simulink model "New_Path_Following_with_Obstacle_Avoidance"  (R2021a)
settings: Solver=FixedStepAuto  StartTime=0.0  StopTime=inf  RelTol=1e-3
undefined symbols (not defined in the file): Angular, Linear, Sonar_Angels, waypoints
libraries: robotlib x5, robotalgslib x2
settings Model: Creator=tarun  LastModifiedBy=tarun
settings OptimizationCC: EnhancedBackFolding=on  PassReuseOutputArgsAs=Individual arguments  ZeroExternalMemoryAtStartup=off  ZeroInternalMemoryAtStartup=off  MaxStackSize=64  OptimizeBlockOrder=speed  DifferentSizesBufferReuse=on  OptimizationCustomize=off  EfficientTunableParamExpr=on
settings DebuggingCC: ParameterTunabilityLossMsg=error
settings HardwareCC: ProdBitPerPointer=32  ProdBitPerSizeT=32  ProdBitPerPtrDiffT=32  ProdLargestAtomicFloat=None  ProdIntDivRoundTo=Undefined  ProdEndianess=Unspecified  ProdWordSize=32  ProdHWDeviceType=Generic->Unspecified (assume 32-bit Generic)
settings SFSimCC: MATLABDynamicMemAlloc=off
settings RTWCC: SystemTargetFile=ert.tlc  HardwareBoard=Robot Operating System (ROS)  TLCOptions="-aInlineSetEventsForThisBaseRateFcn=TLC_FALSE -aSuppressMultiTaskScheduler=TLC_FALSE  -aRateBasedStepFcn=0"  TemplateMakefile=ert_default_tmf  Toolchain=Catkin  TargetLang=C++
settings CodeAppCC: ForceParamTrailComments=on  IgnoreCustomStorageClasses=off  OperatorAnnotations=on  SimulinkDataObjDesc=on  SFDataObjDesc=on  InsertBlockDesc=on
settings ERTTargetCC: SupportVariableSizeSignals=on

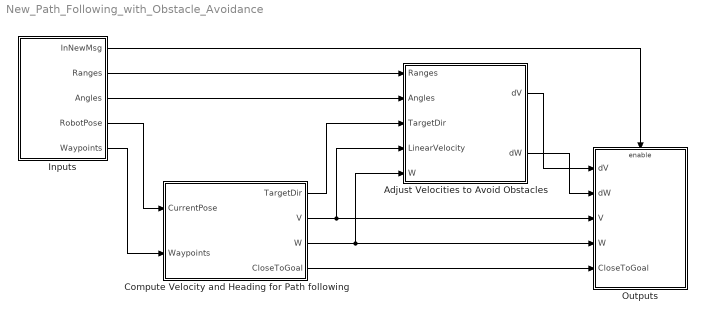
== system New_Path_Following_with_Obstacle_Avoidance ==
  Adjust Velocities to Avoid Obstacles : Subsystem
  Compute Velocity and Heading for Path following : Subsystem
  Inputs : Subsystem
  Outputs : Subsystem
  wires:
  Inputs/1(InNewMsg) -> Outputs/Enable
  Adjust Velocities to Avoid Obstacles/1(dV) -> Outputs/1(dV)
  Inputs/2(Ranges) -> Adjust Velocities to Avoid Obstacles/1(Ranges)
  Compute Velocity and Heading for Path following/1(TargetDir) -> Adjust Velocities to Avoid Obstacles/3(TargetDir)
  Compute Velocity and Heading for Path following/3(W) -> Adjust Velocities to Avoid Obstacles/5(W), Outputs/4(W)
  Compute Velocity and Heading for Path following/2(V) -> Adjust Velocities to Avoid Obstacles/4(LinearVelocity), Outputs/3(V)
  Inputs/5(Waypoints) -> Compute Velocity and Heading for Path following/2(Waypoints)
  Inputs/4(RobotPose) -> Compute Velocity and Heading for Path following/1(CurrentPose)
  Inputs/3(Angles) -> Adjust Velocities to Avoid Obstacles/2(Angles)
  Compute Velocity and Heading for Path following/4(CloseToGoal) -> Outputs/5(CloseToGoal)
  Adjust Velocities to Avoid Obstacles/2(dW) -> Outputs/2(dW)

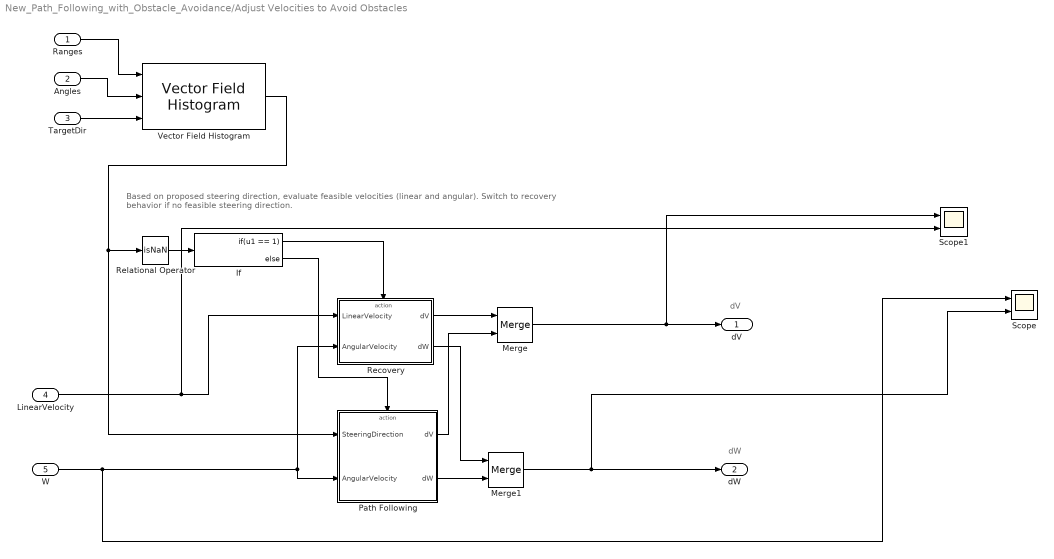
== system New_Path_Following_with_Obstacle_Avoidance/Adjust Velocities to Avoid Obstacles ==
  note: dV
  note: dW
  note: Based on proposed steering direction, evaluate feasible velocities (linear and angular).
      | 				Switch to recovery behavior if no feasible steering direction.
  Ranges : Inport
  Angles : Inport  Port=2
  TargetDir : Inport  Port=3
  LinearVelocity : Inport  Port=4
  W : Inport  Port=5
  If : If  IfExpression=u1 == 1
  Merge : Merge
  Merge1 : Merge
  Path Following : Subsystem  TreatAsAtomicUnit=on
  Recovery : Subsystem  TreatAsAtomicUnit=on
  Relational Operator : RelationalOperator  Operator=isNaN  OutDataTypeStr=boolean  RndMeth=Simplest
  Scope : Scope  NumInputPorts=2
  Scope1 : Scope  NumInputPorts=2
  Vector Field Histogram : robotalgslib/Vector Field Histogram  NumAngularSectors=84  DistanceLimits=[0.2,2]  HistogramThresholds=[1,2]  RobotRadius=0.475  SafetyDistance=0.2  MinTurningRadius=0.2  SimulateUsing=Code generation  TargetDirectionWeight=5  CurrentDirectionWeight=2  PreviousDirectionWeight=2
      settings: SourceProductBaseCode=NV,RO
  dV : Outport
  dW : Outport  Port=2
  wires:
  Angles/1 -> Vector Field Histogram/2
  TargetDir/1 -> Vector Field Histogram/3
  Ranges/1 -> Vector Field Histogram/1
  LinearVelocity/1 -> Scope1/2, Recovery/1(LinearVelocity)
  W/1 -> Scope/1, Path Following/2(AngularVelocity), Recovery/2(AngularVelocity)
  Path Following/1(dV) -> Merge/2
  Recovery/1(dV) -> Merge/1
  Merge/1 -> Scope1/1, dV/1
  Merge1/1 -> Scope/2, dW/1
  If/2 -> Path Following/Action
  Recovery/2(dW) -> Merge1/1
  Relational Operator/1 -> If/1
  If/1 -> Recovery/Action
  Vector Field Histogram/1 -> Path Following/1(SteeringDirection), Relational Operator/1
  Path Following/2(dW) -> Merge1/2

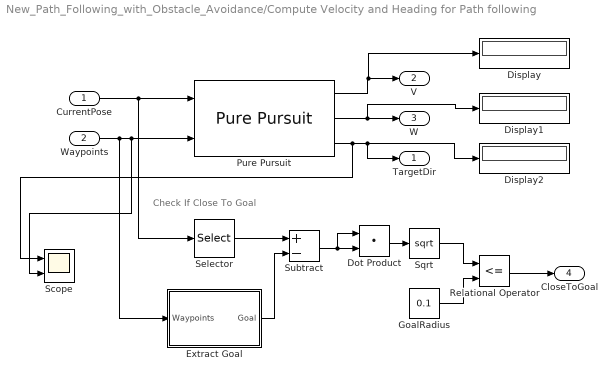
== system New_Path_Following_with_Obstacle_Avoidance/Compute Velocity and Heading for Path following ==
  note: Check If Close To Goal
  CurrentPose : Inport
  Waypoints : Inport  Port=2
  " Extract Goal" : MATLAB Function  TreatAsAtomicUnit=on
  Display : Display
  Display1 : Display
  Display2 : Display
  Dot Product : DotProduct  InputSameDT=on  OutDataTypeStr=Inherit: Inherit via internal rule
  GoalRadius : Constant  Value=0.1
  Pure Pursuit : robotalgslib/Pure Pursuit  DesiredLinearVelocity=0.3  MaxAngularVelocity=0.1  LookaheadDistance=0.45  TargetDirPort=on  SimulateUsing=Code generation
  Relational Operator : RelationalOperator  Operator=<=  OutDataTypeStr=boolean  RndMeth=Simplest
  Scope : Scope  NumInputPorts=2
  Selector : Selector  InputPortWidth=3  IndexOptions=Index vector (dialog)  Indices=[1 2]  OutputSizes=1
  Sqrt : Sqrt  SaturateOnIntegerOverflow=on
  Subtract : Sum  Inputs=+-
  TargetDir : Outport  VectorParamsAs1DForOutWhenUnconnected=off
  V : Outport  Port=2  VectorParamsAs1DForOutWhenUnconnected=off
  W : Outport  Port=3  VectorParamsAs1DForOutWhenUnconnected=off
  CloseToGoal : Outport  Port=4  VectorParamsAs1DForOutWhenUnconnected=off
  wires:
  Pure Pursuit/3 -> Scope/1, Display2/1, TargetDir/1
  Pure Pursuit/2 -> Display1/1, W/1
  Pure Pursuit/1 -> Display/1, V/1
  CurrentPose/1 -> Selector/1, Pure Pursuit/1
  Relational Operator/1 -> CloseToGoal/1
  GoalRadius/1 -> Relational Operator/2
  Selector/1 -> Subtract/1
  Dot Product/1 -> Sqrt/1
  Sqrt/1 -> Relational Operator/1
  Subtract/1 -> Dot Product/1, Dot Product/2
  " Extract Goal"/1(Goal) -> Subtract/2
  Waypoints/1 -> " Extract Goal"/1(Waypoints), Scope/2, Pure Pursuit/2

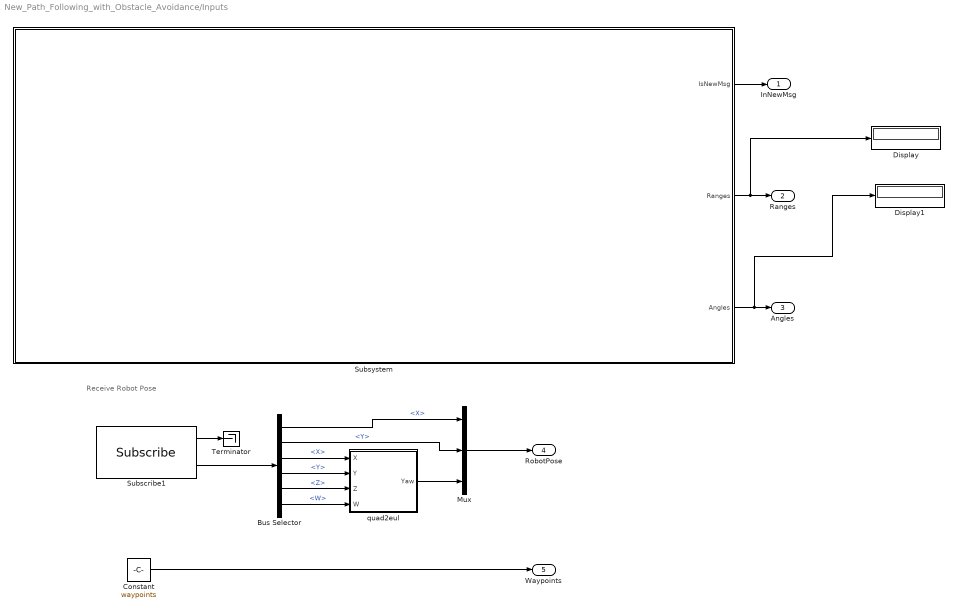
== system New_Path_Following_with_Obstacle_Avoidance/Inputs ==
  note: Receive Robot Pose
  Bus Selector : BusSelector  OutputSignals=Pose.Pose.Position.X,Pose.Pose.Position.Y,Pose.Pose.Orientation.X,Pose.Pose.Orientation.Y,Pose.Pose.Orientation.Z,Pose.Pose.Orientation.W
  Constant : Constant  Value=waypoints
  Display : Display
  Display1 : Display
  Mux : Mux  Inputs=3
  Subscribe1 : robotlib/Subscribe  topicSource=Specify your own  topic=/RosAria/pose  messageType=nav_msgs/Odometry  SampleTime=-1  legacyBusStruct=off  messageQueueLength=1
  Subsystem : Subsystem
  Terminator : Terminator
  quad2eul : MATLAB Function  TreatAsAtomicUnit=on
  InNewMsg : Outport
  Ranges : Outport  Port=2
  Angles : Outport  Port=3
  RobotPose : Outport  Port=4  VectorParamsAs1DForOutWhenUnconnected=off
  Waypoints : Outport  Port=5  VectorParamsAs1DForOutWhenUnconnected=off
  wires:
  quad2eul/1(Yaw) -> Mux/3
  Subscribe1/2 -> Bus Selector/1
  Bus Selector/3 -> quad2eul/1(X)  "<X>"
  Subscribe1/1 -> Terminator/1
  Bus Selector/2 -> Mux/2  "<Y>"
  Bus Selector/5 -> quad2eul/3(Z)  "<Z>"
  Bus Selector/4 -> quad2eul/2(Y)  "<Y>"
  Bus Selector/1 -> Mux/1  "<X>"
  Bus Selector/6 -> quad2eul/4(W)  "<W>"
  Mux/1 -> RobotPose/1
  Subsystem/3(Angles) -> Display1/1, Angles/1
  Subsystem/2(Ranges) -> Display/1, Ranges/1
  Subsystem/1(IsNewMsg) -> InNewMsg/1
  Constant/1 -> Waypoints/1

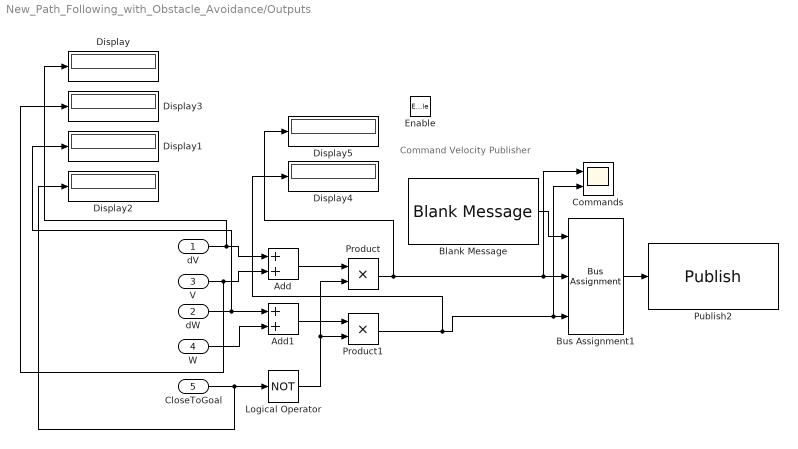
== system New_Path_Following_with_Obstacle_Avoidance/Outputs ==
  note: Command Velocity Publisher
  dV : Inport
  dW : Inport  Port=2
  V : Inport  Port=3
  W : Inport  Port=4
  CloseToGoal : Inport  Port=5
  Enable : EnablePort
  Add : Sum
  Add1 : Sum
  Blank Message : robotlib/Blank Message  messageClass=Message  entityType=geometry_msgs/Twist  messageType=geometry_msgs/Twist  SampleTime=inf  legacyBusStruct=off
  Bus Assignment1 : BusAssignment  DialogController=Simulink.DDGSource_BusAssignment  AssignedSignals=Linear.X,Angular.Z
  Commands : Scope  NumInputPorts=2
  Display{,1..5} (6 alike) : Display
  Logical Operator : Logic  Operator=NOT  AllPortsSameDT=off  OutDataTypeStr=boolean
  Product : Product
  Product1 : Product
  Publish2 : robotlib/Publish  topicSource=Select from ROS network  topic=/RosAria/cmd_vel  messageType=geometry_msgs/Twist  legacyBusStruct=off  messageQueueLength=105
  wires:
  V/1 -> Display3/1, Add/2
  W/1 -> Add1/2
  dV/1 -> Display/1, Add/1
  dW/1 -> Display1/1, Add1/1
  CloseToGoal/1 -> Display2/1, Logical Operator/1
  Add/1 -> Product/1
  Add1/1 -> Product1/1
  Product/1 -> Display5/1, Bus Assignment1/2, Commands/1
  Blank Message/1 -> Bus Assignment1/1
  Bus Assignment1/1 -> Publish2/1
  Logical Operator/1 -> Product1/2, Product/2
  Product1/1 -> Display4/1, Commands/2, Bus Assignment1/3

== system New_Path_Following_with_Obstacle_Avoidance/Adjust Velocities to Avoid Obstacles/Path Following ==
  SteeringDirection : Inport
  AngularVelocity : Inport  Port=2
  Action Port : ActionPort  ActionPortLabel=else
  Compute Angular Velocity : MATLAB Function  TreatAsAtomicUnit=on
  Constant : Constant  Value=0
  MaxAngularVelocity : Constant
  Subtract : Sum  Inputs=+-
  dV : Outport  VectorParamsAs1DForOutWhenUnconnected=off
  dW : Outport  Port=2  VectorParamsAs1DForOutWhenUnconnected=off
  wires:
  Constant/1 -> dV/1
  MaxAngularVelocity/1 -> Compute Angular Velocity/2(wMax)
  SteeringDirection/1 -> Compute Angular Velocity/1(steeringDir)
  Subtract/1 -> dW/1
  Compute Angular Velocity/1(w) -> Subtract/1
  AngularVelocity/1 -> Subtract/2

== system New_Path_Following_with_Obstacle_Avoidance/Adjust Velocities to Avoid Obstacles/Recovery ==
  LinearVelocity : Inport
  AngularVelocity : Inport  Port=2
  Action Port : ActionPort  ActionPortLabel=if(u1 == 1)
  Constant1 : Constant  Value=0.2
  Gain : Gain  Gain=-1
  Subtract : Sum  Inputs=+-
  dV : Outport  VectorParamsAs1DForOutWhenUnconnected=off
  dW : Outport  Port=2  VectorParamsAs1DForOutWhenUnconnected=off
  wires:
  LinearVelocity/1 -> Gain/1
  Gain/1 -> dV/1
  Constant1/1 -> Subtract/1
  AngularVelocity/1 -> Subtract/2
  Subtract/1 -> dW/1

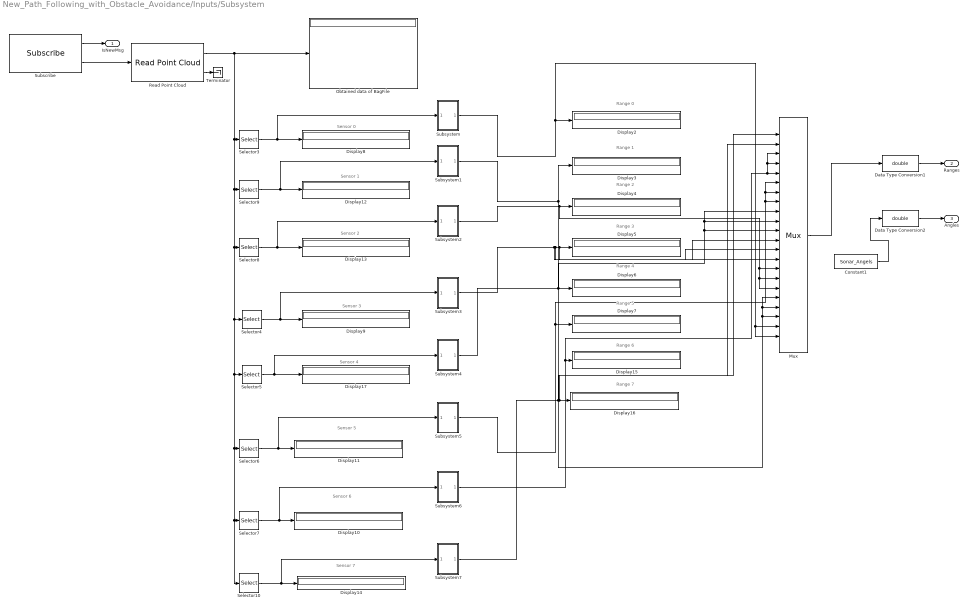
== system New_Path_Following_with_Obstacle_Avoidance/Inputs/Subsystem ==
  note: Range 7
  note: Range 4
  note: Sensor 2
  note: Range 2
  note: Sensor 3
  note: Sensor 1
  note: Range 3
  note: Sensor 6
  note: Range 5
  note: Range 0
  note: Sensor 0
  note: Sensor 4
  note: Sensor 5
  note: Range 1
  note: Range 6
  note: Sensor 7
  Constant1 : Constant  Value=Sonar_Angels
  Data Type Conversion1 : DataTypeConversion  OutDataTypeStr=double
  Data Type Conversion2 : DataTypeConversion  OutDataTypeStr=double
  Display{2..17} (16 alike) : Display
  Mux : Mux  Inputs=22
  Obtained data of BagFile : Display
  Read Point Cloud : robotlib/Read Point Cloud  MaximumPointCloudSize=[8, 1]  PreserveStructure=off  ShowRGBOutput=off  ShowIntensityOutput=off  ShowErrorCodeOutput=on  VariableSizeOutputs=off
      settings: SourceProductBaseCode=RR
  Selector10 : Selector  NumberOfDimensions=2  InputPortWidth=6  IndexOptions=Starting index (dialog),Starting index (dialog)  Indices=8,1  OutputSizes=1,3
  Selector3 : Selector  NumberOfDimensions=2  InputPortWidth=6  IndexOptions=Starting index (dialog),Starting index (dialog)  Indices=1,1  OutputSizes=1,3
  Selector4 : Selector  NumberOfDimensions=2  InputPortWidth=6  IndexOptions=Starting index (dialog),Starting index (dialog)  Indices=4,1  OutputSizes=1,3
  Selector5 : Selector  NumberOfDimensions=2  InputPortWidth=6  IndexOptions=Starting index (dialog),Starting index (dialog)  Indices=5,1  OutputSizes=1,3
  Selector6 : Selector  NumberOfDimensions=2  InputPortWidth=6  IndexOptions=Starting index (dialog),Starting index (dialog)  Indices=6,1  OutputSizes=1,3
  Selector7 : Selector  NumberOfDimensions=2  InputPortWidth=6  IndexOptions=Starting index (dialog),Starting index (dialog)  Indices=7,1  OutputSizes=1,3
  Selector8 : Selector  NumberOfDimensions=2  InputPortWidth=6  IndexOptions=Starting index (dialog),Starting index (dialog)  Indices=3,1  OutputSizes=1,3
  Selector9 : Selector  NumberOfDimensions=2  InputPortWidth=6  IndexOptions=Starting index (dialog),Starting index (dialog)  Indices=2,1  OutputSizes=1,3
  Subscribe : robotlib/Subscribe  topicSource=Select from ROS network  topic=/RosAria/sonar_pointcloud2  messageType=sensor_msgs/PointCloud2  SampleTime=0.05  legacyBusStruct=off  messageQueueLength=1
  Subsystem : Subsystem
  Subsystem1 : Subsystem
  Subsystem2 : Subsystem
  Subsystem3 : Subsystem
  Subsystem4 : Subsystem
  Subsystem5 : Subsystem
  Subsystem6 : Subsystem
  Subsystem7 : Subsystem
  Terminator : Terminator
  IsNewMsg : Outport
  Ranges : Outport  Port=2
  Angles : Outport  Port=3
  wires:
  Mux/1 -> Data Type Conversion1/1
  Constant1/1 -> Data Type Conversion2/1
  Selector4/1 -> Subsystem3/1(In1), Display9/1
  Subsystem7/1(Out1) -> Mux/2, Mux/1, Display16/1
  Selector8/1 -> Subsystem2/1(In1), Display13/1
  Subsystem5/1(Out1) -> Mux/6, Mux/7, Mux/8, Display7/1
  Selector9/1 -> Subsystem1/1(In1), Display12/1
  Subsystem2/1(Out1) -> Mux/17, Mux/16, Mux/15, Display4/1
  Selector3/1 -> Subsystem/1(In1), Display8/1
  Subsystem6/1(Out1) -> Mux/4, Mux/3, Mux/5, Display15/1
  Read Point Cloud/2 -> Terminator/1
  Subsystem4/1(Out1) -> Mux/9, Mux/10, Mux/11, Display6/1
  Selector6/1 -> Subsystem5/1(In1), Display11/1
  Subsystem1/1(Out1) -> Mux/20, Mux/19, Mux/18, Display3/1
  Subsystem/1(Out1) -> Mux/22, Mux/21, Display2/1
  Selector5/1 -> Subsystem4/1(In1), Display17/1
  Selector10/1 -> Subsystem7/1(In1), Display14/1
  Subsystem3/1(Out1) -> Mux/13, Mux/12, Mux/14, Display5/1
  Selector7/1 -> Subsystem6/1(In1), Display10/1
  Subscribe/2 -> Read Point Cloud/1
  Read Point Cloud/1 -> Obtained data of BagFile/1, Selector3/1, Selector9/1, Selector8/1, Selector4/1, Selector5/1, Selector6/1, Selector10/1, Selector7/1
  Subscribe/1 -> IsNewMsg/1
  Data Type Conversion1/1 -> Ranges/1
  Data Type Conversion2/1 -> Angles/1

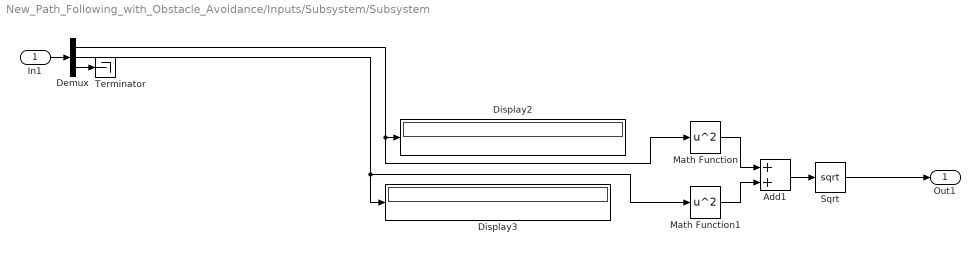
== system New_Path_Following_with_Obstacle_Avoidance/Inputs/Subsystem/Subsystem ==
  In1 : Inport
  Add1 : Sum
  Demux : Demux  Outputs=3
  Display2 : Display
  Display3 : Display
  Math Function : Math  Operator=square  SaturateOnIntegerOverflow=on
  Math Function1 : Math  Operator=square  SaturateOnIntegerOverflow=on
  Sqrt : Sqrt  SaturateOnIntegerOverflow=on
  Terminator : Terminator
  Out1 : Outport
  wires:
  Math Function1/1 -> Add1/2
  Demux/1 -> Math Function/1, Display2/1
  In1/1 -> Demux/1
  Math Function/1 -> Add1/1
  Demux/2 -> Display3/1, Math Function1/1
  Sqrt/1 -> Out1/1
  Add1/1 -> Sqrt/1
  Demux/3 -> Terminator/1

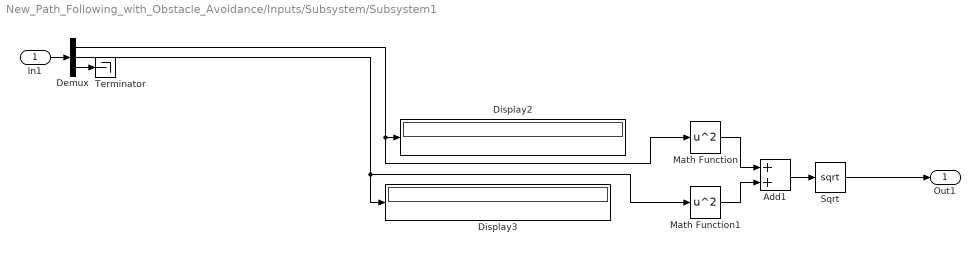
== system New_Path_Following_with_Obstacle_Avoidance/Inputs/Subsystem/Subsystem1 ==
  In1 : Inport
  Add1 : Sum
  Demux : Demux  Outputs=3
  Display2 : Display
  Display3 : Display
  Math Function : Math  Operator=square  SaturateOnIntegerOverflow=on
  Math Function1 : Math  Operator=square  SaturateOnIntegerOverflow=on
  Sqrt : Sqrt  SaturateOnIntegerOverflow=on
  Terminator : Terminator
  Out1 : Outport
  wires:
  Math Function1/1 -> Add1/2
  Demux/1 -> Math Function/1, Display2/1
  In1/1 -> Demux/1
  Math Function/1 -> Add1/1
  Demux/2 -> Display3/1, Math Function1/1
  Sqrt/1 -> Out1/1
  Add1/1 -> Sqrt/1
  Demux/3 -> Terminator/1

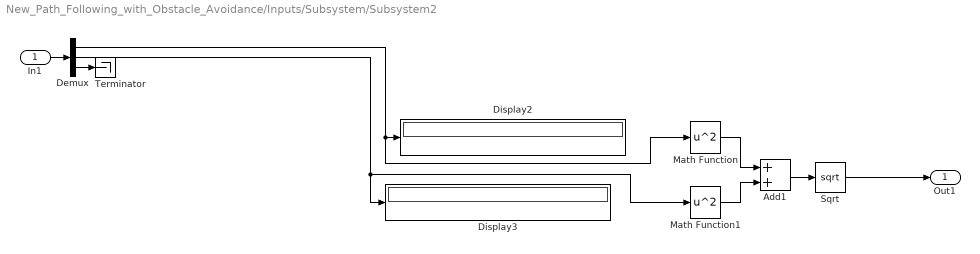
== system New_Path_Following_with_Obstacle_Avoidance/Inputs/Subsystem/Subsystem2 ==
  In1 : Inport
  Add1 : Sum
  Demux : Demux  Outputs=3
  Display2 : Display
  Display3 : Display
  Math Function : Math  Operator=square  SaturateOnIntegerOverflow=on
  Math Function1 : Math  Operator=square  SaturateOnIntegerOverflow=on
  Sqrt : Sqrt  SaturateOnIntegerOverflow=on
  Terminator : Terminator
  Out1 : Outport
  wires:
  Math Function1/1 -> Add1/2
  Demux/1 -> Math Function/1, Display2/1
  In1/1 -> Demux/1
  Math Function/1 -> Add1/1
  Demux/2 -> Display3/1, Math Function1/1
  Sqrt/1 -> Out1/1
  Add1/1 -> Sqrt/1
  Demux/3 -> Terminator/1

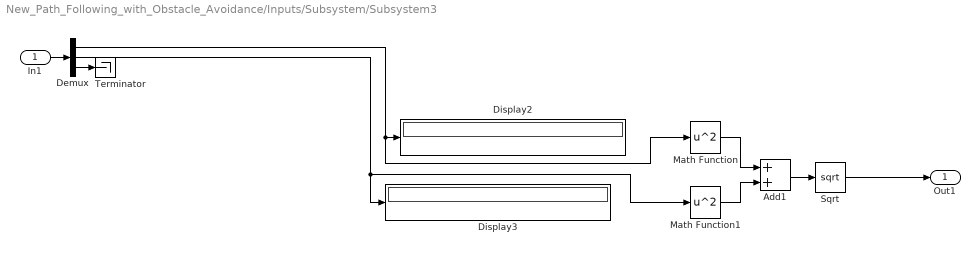
== system New_Path_Following_with_Obstacle_Avoidance/Inputs/Subsystem/Subsystem3 ==
  In1 : Inport
  Add1 : Sum
  Demux : Demux  Outputs=3
  Display2 : Display
  Display3 : Display
  Math Function : Math  Operator=square  SaturateOnIntegerOverflow=on
  Math Function1 : Math  Operator=square  SaturateOnIntegerOverflow=on
  Sqrt : Sqrt  SaturateOnIntegerOverflow=on
  Terminator : Terminator
  Out1 : Outport
  wires:
  Math Function1/1 -> Add1/2
  Demux/1 -> Math Function/1, Display2/1
  In1/1 -> Demux/1
  Math Function/1 -> Add1/1
  Demux/2 -> Display3/1, Math Function1/1
  Sqrt/1 -> Out1/1
  Add1/1 -> Sqrt/1
  Demux/3 -> Terminator/1

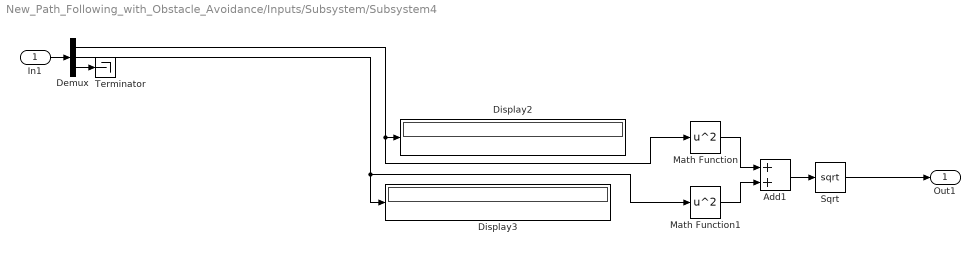
== system New_Path_Following_with_Obstacle_Avoidance/Inputs/Subsystem/Subsystem4 ==
  In1 : Inport
  Add1 : Sum
  Demux : Demux  Outputs=3
  Display2 : Display
  Display3 : Display
  Math Function : Math  Operator=square  SaturateOnIntegerOverflow=on
  Math Function1 : Math  Operator=square  SaturateOnIntegerOverflow=on
  Sqrt : Sqrt  SaturateOnIntegerOverflow=on
  Terminator : Terminator
  Out1 : Outport
  wires:
  Math Function1/1 -> Add1/2
  Demux/1 -> Math Function/1, Display2/1
  In1/1 -> Demux/1
  Math Function/1 -> Add1/1
  Demux/2 -> Display3/1, Math Function1/1
  Sqrt/1 -> Out1/1
  Add1/1 -> Sqrt/1
  Demux/3 -> Terminator/1

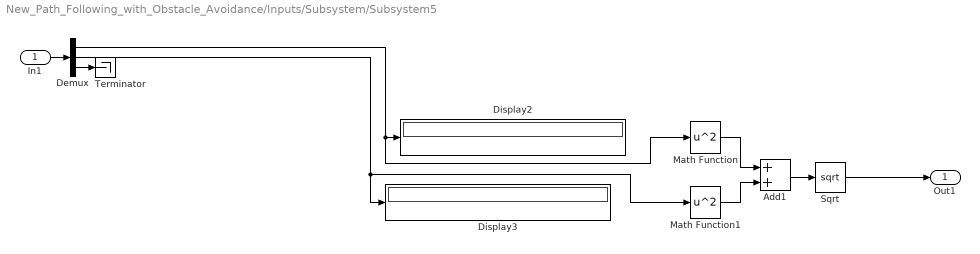
== system New_Path_Following_with_Obstacle_Avoidance/Inputs/Subsystem/Subsystem5 ==
  In1 : Inport
  Add1 : Sum
  Demux : Demux  Outputs=3
  Display2 : Display
  Display3 : Display
  Math Function : Math  Operator=square  SaturateOnIntegerOverflow=on
  Math Function1 : Math  Operator=square  SaturateOnIntegerOverflow=on
  Sqrt : Sqrt  SaturateOnIntegerOverflow=on
  Terminator : Terminator
  Out1 : Outport
  wires:
  Math Function1/1 -> Add1/2
  Demux/1 -> Math Function/1, Display2/1
  In1/1 -> Demux/1
  Math Function/1 -> Add1/1
  Demux/2 -> Display3/1, Math Function1/1
  Sqrt/1 -> Out1/1
  Add1/1 -> Sqrt/1
  Demux/3 -> Terminator/1

== system New_Path_Following_with_Obstacle_Avoidance/Inputs/Subsystem/Subsystem6 ==
  In1 : Inport
  Add1 : Sum
  Demux : Demux  Outputs=3
  Display2 : Display
  Display3 : Display
  Math Function : Math  Operator=square  SaturateOnIntegerOverflow=on
  Math Function1 : Math  Operator=square  SaturateOnIntegerOverflow=on
  Sqrt : Sqrt  SaturateOnIntegerOverflow=on
  Terminator : Terminator
  Out1 : Outport
  wires:
  Math Function1/1 -> Add1/2
  Demux/1 -> Math Function/1, Display2/1
  In1/1 -> Demux/1
  Math Function/1 -> Add1/1
  Demux/2 -> Display3/1, Math Function1/1
  Sqrt/1 -> Out1/1
  Add1/1 -> Sqrt/1
  Demux/3 -> Terminator/1

== system New_Path_Following_with_Obstacle_Avoidance/Inputs/Subsystem/Subsystem7 ==
  In1 : Inport
  Add1 : Sum
  Demux : Demux  Outputs=3
  Display2 : Display
  Display3 : Display
  Math Function : Math  Operator=square  SaturateOnIntegerOverflow=on
  Math Function1 : Math  Operator=square  SaturateOnIntegerOverflow=on
  Sqrt : Sqrt  SaturateOnIntegerOverflow=on
  Terminator : Terminator
  Out1 : Outport
  wires:
  Math Function1/1 -> Add1/2
  Demux/1 -> Math Function/1, Display2/1
  In1/1 -> Demux/1
  Math Function/1 -> Add1/1
  Demux/2 -> Display3/1, Math Function1/1
  Sqrt/1 -> Out1/1
  Add1/1 -> Sqrt/1
  Demux/3 -> Terminator/1

== matlab function New_Path_Following_with_Obstacle_Avoidance/Inputs/quad2eul ==
  data: X input; Yaw output; Y input; Z input; W input
function Yaw = quat2eulBlk(X, Y, Z, W)
%#codegen

eularAngles = quat2eul([W, X, Y, Z]);
Yaw = eularAngles(1);

== matlab function New_Path_Following_with_Obstacle_Avoidance/Compute Velocity and Heading for Path following/ Extract Goal ==
  data: Waypoints input; Goal output
function Goal = extractGoal(Waypoints)
%#codegen
b = isnan(Waypoints);
[rows,~] = find(b);
ridx = setdiff(1:size(Waypoints,1), sort(rows));
Goal = [Waypoints(ridx(end), 1) Waypoints(ridx(end), 2)];

== matlab function New_Path_Following_with_Obstacle_Avoidance/Adjust Velocities to Avoid Obstacles/Path Following/Compute Angular Velocity ==
  data: steeringDir input; w output; wMax input
function w = exampleHelperComputeAngularVelocity(steeringDir, wMax)
%EXAMPLEHELPERCOMPUTEANGULARVELOCITY Compute angular velocity
%   W = exampleHelperComputeAngularVelocity(STEERINGDIR)
%   returns the angular velocity W for a differential drive robot in radians
%   per second for a given steering direction STEERINGDIR in the robot's
%   coordinate frame in radians.
%
%   W = exampleHelperComputeAngularVelocity(STEERINGDIR, WMAX)
%   returns the angular velocity W for a differential drive robot in radians
%   per second for a given steering direction STEERINGDIR in the robot's
%   coordinate frame in radians and maximum angular velocity WMAX in
%   radians per second. The output angular velocity is saturated based on
%   the WMAX.
%
%   Example:
%       
%       w = exampleHelperComputeAngularVelocity(0.2, 1);

% Copyright 2015 The MathWorks, Inc.

%#codegen
%#ok<*EMCA>

% Allow variable input arguments
if nargin == 1   
    wMax = inf;
end

validateattributes(steeringDir, {'double'},{'real'},...
    'exampleHelperComputeAngularVelocity', 'STEERINGDIR', 1);
validateattributes(wMax, {'double'},{'real', 'positive'},...
    'exampleHelperComputeAngularVelocity', 'WMAX', 2);

% Computing in robot's coordinate frame
curPose = [0 0 0];

% The following computation is similar to robotics.PurePursuit
lookaheadPoint = [cos(steeringDir), sin(steeringDir)];
slope = atan2((lookaheadPoint(2) - curPose(2)), ...
    (lookaheadPoint(1) - curPose(1)));
alpha = angdiff(curPose(3), slope);

% Angular velocity command for a differential drive robot is
% equal to the desired curvature to be followed by the robot.

w = (2*sin(alpha));

% Pick a constant rotation when robot is facing in the opposite
% direction of the path
if abs(abs(alpha) - pi) < 1e-12
    w = sign(w)*1;
end

if abs(w) > wMax
    w = sign(w)*wMax;
end

end
